simulink model "SCBI_for_Costant_DC"  (R2018a)
settings: Solver=ode23t  StartTime=0.0  StopTime=.2  MaxStep=1e-6  RelTol=1e-3
libraries: powerlib x22, simulink x4, dspstat3 x1
settings Model: Creator=asus  LastModifiedBy=asus

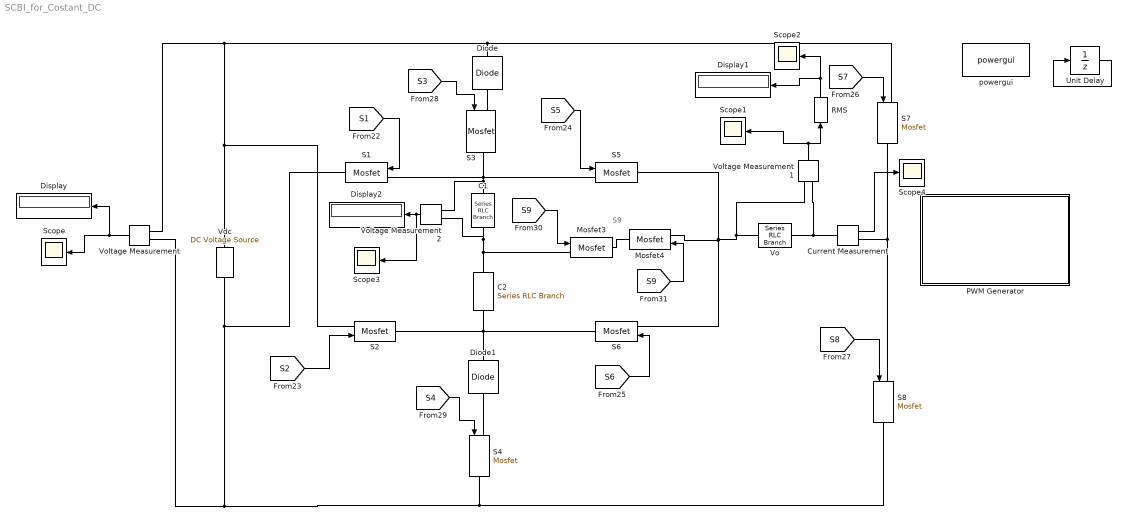
== system SCBI_for_Costant_DC ==
  note: S9
  C1 : powerlib/Elements/Series RLC Branch  LConnTagsString=__new0  RConnTagsString=__new0  BranchType=C  Resistance=1  Inductance=1e-3  SetiL0=off  InitialCurrent=0  Capacitance=1000e-6  Setx0=off  InitialVoltage=0  Measurements=None
  C2 : powerlib/Elements/Series RLC Branch  LConnTagsString=__new0  RConnTagsString=__new0  BranchType=C  Resistance=1  Inductance=1e-3  SetiL0=off  InitialCurrent=0  Capacitance=1000e-6  Setx0=off  InitialVoltage=0  Measurements=None
  Current Measurement : powerlib/Measurements/Current Measurement  PhasorSimulation=off  OutputType=Complex  PSBequivalent=0
  Diode : powerlib/Power Electronics/Diode  Ron=0.001  Lon=0  Vf=0.8  IC=0  UseSnubber=0  Rs=500  Cs=250e-9  Measurements=off
  Diode1 : powerlib/Power Electronics/Diode  Ron=0.001  Lon=0  Vf=0.8  IC=0  UseSnubber=0  Rs=500  Cs=250e-9  Measurements=off
  Display : Display
  Display1 : Display
  Display2 : Display
  Mosfet3 : powerlib/Power Electronics/Mosfet  Ron=0.1  Lon=0  Rd=0.01  Vfd=0  IC=0  Rs=1e5  Cs=inf  Measurements=off
  Mosfet4 : powerlib/Power Electronics/Mosfet  Ron=0.1  Lon=0  Rd=0.01  Vfd=0  IC=0  Rs=1e5  Cs=inf  Measurements=off
  PWM Generator : Subsystem
  RMS : dspstat3/RMS  run=off  directionMode=Each column  dimension=1  InputProcessing=Columns as channels (frame based)  reset_popup=None
  S{1,3,5..8} (6 alike) : powerlib/Power Electronics/Mosfet  Ron=0.1  Lon=0  Rd=0.01  Vfd=0  IC=0  Rs=1e5  Cs=inf  Measurements=off
  "S2 " : powerlib/Power Electronics/Mosfet  Ron=0.1  Lon=0  Rd=0.01  Vfd=0  IC=0  Rs=1e5  Cs=inf  Measurements=off
  "S4 " : powerlib/Power Electronics/Mosfet  Ron=0.1  Lon=0  Rd=0.01  Vfd=0  IC=0  Rs=1e5  Cs=inf  Measurements=off
  Scope{,1..4} (5 alike) : Scope
  Unit Delay : UnitDelay  SampleTime=0.0001
  Vdc : powerlib/Electrical Sources/DC Voltage Source  Amplitude=183  Measurements=None
  Vo : powerlib/Elements/Series RLC Branch  LConnTagsString=__new0  RConnTagsString=__new0  BranchType=R  Resistance=110  Inductance=50e-3  SetiL0=off  InitialCurrent=0  Capacitance=1e-6  Setx0=off  InitialVoltage=0  Measurements=None
  Voltage Measurement : powerlib/Measurements/Voltage Measurement  PhasorSimulation=off  OutputType=Complex  PSBequivalent=0
  Voltage Measurement1 : powerlib/Measurements/Voltage Measurement  PhasorSimulation=off  OutputType=Complex  PSBequivalent=0
  Voltage Measurement2 : powerlib/Measurements/Voltage Measurement  PhasorSimulation=off  OutputType=Complex  PSBequivalent=0
  powergui : powerlib/powergui  Priority=1  SimulationMode=Continuous  SampleTime=50e-6  frequency=60  Iterations=50  frequencyindice=0  Pbase=100e6  ErrMax=1e-4  UnitsV=kV  UnitsW=MW  buscounter=0  FunctionMessages=off  echomessages=off  EnableUseOfTLC=off  CurrentSourceSwitches=off  DisableSnubberDevices=off  DisableRonSwitches=off  DisableVfSwitches=off  DisplayEquations=off  SolverType=Tustin/Backward Euler (TBE)  Interpol=off  ExternalGateDelay=off  methode=off  Ts=100  x0status=blocks  SPID=on  SwTol=0  HookPort=off  RestoreLinks=warning  ResistiveCurrentMeasurement=off  Frange=[0:2:500]  Ylog=off  Xlog=on  ShowGrid=off  save=off  variable=ZData  structure=Io  ZoomFFT=off  StartTime=0.0  cycles=5  DisplayStyle=1  fundamental=50  FreqAxis=off  MaxFrequency=1000  frequencyindicesteady=1  RmsSteady=1  display=off
  wires:
  [S1] -> S1/1
  [S5] -> S5/1
  [S2] -> "S2 "/1
  [S6] -> S6/1
  [S8] -> S8/1
  [S7] -> S7/1
  [S3] -> S3/1
  [S4] -> "S4 "/1
  [S9] -> Mosfet3/1
  [S9] -> Mosfet4/1
  Voltage Measurement/1 -> Scope/1, Display/1
  Voltage Measurement1/1 -> Scope1/1, RMS/1
  Unit Delay/1 -> Unit Delay/1
  Voltage Measurement2/1 -> Scope3/1, Display2/1
  RMS/1 -> Display1/1, Scope2/1
  Current Measurement/1 -> Scope4/1
  connections:
  Diode/RConn1 -- S3/LConn1
  Diode/LConn1 -- Voltage Measurement/LConn1 -- Vdc/RConn1 -- "S2 "/LConn1 -- S7/LConn1
  C1/LConn1 -- Voltage Measurement2/LConn1 -- S5/LConn1 -- S3/RConn1 -- S1/LConn1
  Mosfet3/LConn1 -- Voltage Measurement2/LConn2 -- C1/RConn1 -- C2/LConn1
  C2/RConn1 -- "S2 "/RConn1 -- Diode1/LConn1 -- S6/RConn1
  S8/RConn1 -- "S4 "/RConn1 -- Vdc/LConn1 -- S1/RConn1 -- Voltage Measurement/LConn2
  Mosfet4/RConn1 -- Mosfet3/RConn1
  Vo/LConn1 -- Voltage Measurement1/LConn1 -- S5/RConn1 -- Mosfet4/LConn1 -- S6/LConn1
  Voltage Measurement1/LConn2 -- Current Measurement/LConn1 -- Vo/RConn1
  Diode1/RConn1 -- "S4 "/LConn1
  S7/RConn1 -- Current Measurement/RConn1 -- S8/LConn1

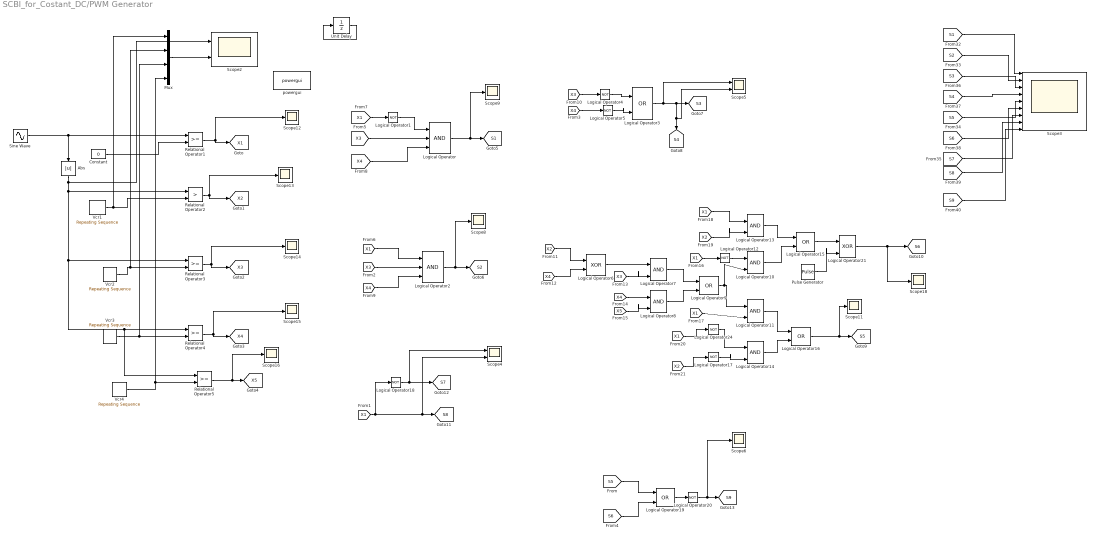
== system SCBI_for_Costant_DC/PWM Generator ==
  Abs : Abs
  Constant : Constant  Value=0
  Logical Operator : Logic  Inputs=3  IconShape=distinctive  AllPortsSameDT=off  OutDataTypeStr=boolean
  Logical Operator{1,4..5,12,17..18,20,24} (8 alike) : Logic  Operator=NOT  Inputs=3  IconShape=distinctive  AllPortsSameDT=off  OutDataTypeStr=boolean
  Logical Operator{7..8,10..11,13..14} (6 alike) : Logic  IconShape=distinctive  AllPortsSameDT=off  OutDataTypeStr=boolean
  Logical Operator{3,9,15..16,19} (5 alike) : Logic  Operator=OR  IconShape=distinctive  AllPortsSameDT=off  OutDataTypeStr=boolean
  Logical Operator2 : Logic  Inputs=3  IconShape=distinctive  AllPortsSameDT=off  OutDataTypeStr=boolean
  Logical Operator21 : Logic  Operator=XOR  IconShape=distinctive  AllPortsSameDT=off  OutDataTypeStr=boolean
  Logical Operator6 : Logic  Operator=XOR  IconShape=distinctive  AllPortsSameDT=off  OutDataTypeStr=boolean
  Mux : Mux
  Pulse Generator : DiscretePulseGenerator  PulseType=Time based  Period=0.02  PulseWidth=50
  Relational Operator{1,3..5} (4 alike) : RelationalOperator  OutDataTypeStr=boolean  RndMeth=Simplest
  Relational Operator2 : RelationalOperator  Operator=>  OutDataTypeStr=boolean  RndMeth=Simplest
  Scope{6,8..9,11..16,18} (10 alike) : Scope
  Scope2 : Scope  NumInputPorts=2
  Scope3 : Scope  NumInputPorts=9
  Scope4 : Scope  NumInputPorts=2
  Scope5 : Scope  NumInputPorts=2
  Sine Wave : Sin  Amplitude=3.9  Frequency=2*pi*50  SampleTime=1e-6
  Unit Delay : UnitDelay  SampleTime=-1
  Vcr1 : simulink/Sources/Repeating Sequence  rep_seq_t=[0 0.0002 0.0004]  rep_seq_y=[0 1 0]
  Vcr2 : simulink/Sources/Repeating Sequence  rep_seq_t=[0 0.0002 0.0004]  rep_seq_y=[1 2 1]
  Vcr3 : simulink/Sources/Repeating Sequence  rep_seq_t=[0 0.0002 0.0004]  rep_seq_y=[2 3 2]
  Vcr4 : simulink/Sources/Repeating Sequence  rep_seq_t=[0 0.0002 0.0004]  rep_seq_y=[3 4 3]
  powergui : powerlib/powergui  Priority=1  SimulationMode=Continuous  SampleTime=50e-6  frequency=60  Iterations=50  frequencyindice=0  Pbase=100e6  ErrMax=1e-4  UnitsV=kV  UnitsW=MW  buscounter=0  FunctionMessages=off  echomessages=off  EnableUseOfTLC=off  CurrentSourceSwitches=off  DisableSnubberDevices=off  DisableRonSwitches=off  DisableVfSwitches=off  DisplayEquations=off  SolverType=Tustin/Backward Euler (TBE)  Interpol=off  ExternalGateDelay=off  methode=off  Ts=100  x0status=blocks  SPID=on  SwTol=0  HookPort=off  RestoreLinks=warning  ResistiveCurrentMeasurement=off  Frange=[0:2:500]  Ylog=off  Xlog=on  ShowGrid=off  save=off  variable=ZData  structure=0  ZoomFFT=off  StartTime=0.0  cycles=1  DisplayStyle=1  fundamental=60  FreqAxis=off  MaxFrequency=1000  frequencyindicesteady=1  RmsSteady=1  display=off
  tag scope: S1=global, S2=global, S3=global, S4=global, S5=global, S6=global, S7=global, S8=global, S9=global, X1=global, X2=global, X3=global, X4=global, X5=global
  wires:
  Vcr4/1 -> Mux/4, Relational Operator5/2
  Relational Operator3/1 -> [X3], Scope14/1
  [X3] -> Logical Operator4/1
  [S9] -> Scope3/9
  Logical Operator10/1 -> Logical Operator15/2
  [X3] -> Logical Operator7/2
  Relational Operator2/1 -> [X2], Scope13/1
  Vcr2/1 -> Mux/2, Relational Operator3/2
  [S6] -> Scope3/6
  Constant/1 -> Relational Operator1/2
  [X3] -> Logical Operator/2
  Relational Operator1/1 -> [X1], Scope12/1
  Relational Operator5/1 -> [X5], Scope16/1
  [X1] -> Logical Operator12/1
  Vcr1/1 -> Mux/1, Relational Operator2/2
  Logical Operator5/1 -> Logical Operator3/2
  [X4] -> Logical Operator/3
  [S3] -> Scope3/3
  Logical Operator3/1 -> Scope5/1, Scope5/2, [S4], [S3]
  Logical Operator19/1 -> Logical Operator20/1
  [S7] -> Scope3/7
  Abs/1 -> Scope2/1, Relational Operator2/1, Relational Operator3/1, Relational Operator4/1, Relational Operator5/1
  [S2] -> Scope3/2
  [S4] -> Scope3/4
  [X3] -> Logical Operator2/2
  Unit Delay/1 -> Unit Delay/1
  Vcr3/1 -> Mux/3, Relational Operator4/2
  Logical Operator13/1 -> Logical Operator15/1
  Logical Operator15/1 -> Logical Operator21/1
  [X4] -> Logical Operator5/1
  [X1] -> Logical Operator2/1
  Mux/1 -> Scope2/2
  [S1] -> Scope3/1
  [X2] -> Logical Operator17/1
  Relational Operator4/1 -> [X4], Scope15/1
  [X5] -> Logical Operator8/2
  [S8] -> Scope3/8
  [X4] -> Logical Operator8/1
  [X4] -> Logical Operator2/3
  Sine Wave/1 -> Abs/1, Relational Operator1/1
  Logical Operator6/1 -> Logical Operator7/1
  Logical Operator9/1 -> Logical Operator11/1, Logical Operator10/2
  [X1] -> Logical Operator18/1, Scope4/2, [S8]
  [S5] -> Scope3/5
  [X2] -> Logical Operator6/1
  Logical Operator1/1 -> Logical Operator/1
  [S5] -> Logical Operator19/1
  [X1] -> Logical Operator24/1
  Logical Operator14/1 -> Logical Operator16/2
  [S6] -> Logical Operator19/2
  Logical Operator4/1 -> Logical Operator3/1
  Logical Operator18/1 -> Scope4/1, [S7]
  Logical Operator11/1 -> Logical Operator16/1
  Logical Operator20/1 -> Scope6/1, [S9]
  Logical Operator12/1 -> Logical Operator10/1
  Logical Operator7/1 -> Logical Operator9/1
  Logical Operator8/1 -> Logical Operator9/2
  Logical Operator16/1 -> [S5], Scope11/1
  Logical Operator17/1 -> Logical Operator14/2
  [X1] -> Logical Operator11/2
  [X1] -> Logical Operator13/1
  Logical Operator/1 -> Scope9/1, [S1]
  Logical Operator2/1 -> Scope8/1, [S2]
  [X2] -> Logical Operator13/2
  Pulse Generator/1 -> Logical Operator21/2
  [X1] -> Logical Operator1/1
  [X4] -> Logical Operator6/2
  Logical Operator21/1 -> Scope18/1, [S6]
  Logical Operator24/1 -> Logical Operator14/1
